simulink model "pato4CM00_plantModel"  (R2017b)
settings: Solver=FixedStepDiscrete  StartTime=0.0  StopTime=1.8  FixedStep=1/2048  RelTol=1e-3  EnableMultiTasking=on
settings Model: ExtModeAutoUpdateStatusClock=off  Creator=root  LastModifiedBy=Job
settings DataIOCC: SaveFormat=Array  SignalLoggingSaveFormat=ModelDataLogs
settings OptimizationCC: ExpressionDepthLimit=2147483647  InitFltsAndDblsToZero=on  LifeSpan=inf
settings DebuggingCC: UnderspecifiedInitializationDetection=Classic  MergeDetectMultiDrivingBlocksExec=none  SolverPrmCheckMsg=warning  FcnCallInpInsideContextMsg=warning  AllowSymbolicDim=off  StateNameClashWarn=warning  SFUnexpectedBacktrackingDiag=warning  SFNoUnconditionalDefaultTransitionDiag=warning  SFExecutionAtInitializationDiag=none
settings HardwareCC: ProdBitPerPointer=32  ProdBitPerSizeT=32  ProdBitPerPtrDiffT=32  ProdLargestAtomicFloat=None  ProdIntDivRoundTo=Undefined  ProdEndianess=Unspecified  ProdWordSize=32  ProdHWDeviceType=32-bit Generic
settings ModelReferenceCC: PropagateSignalLabelsOutOfModel=off
settings RTWCC: SystemTargetFile=ectarget.tlc  MakeCommand="make_rtw OPTS=\"-DNETIF_ID=2\""  TemplateMakefile=ec_unix.tmf  Description=EtherCAT Real-Time Target for SOEM (IME Technologies 2008)
settings CodeAppCC: StateflowObjectComments=on
settings GRTTargetCC: TargetLangStandard=C89/C90 (ANSI)  GeneratePreprocessorConditionals=Disable all  CombineOutputUpdateFcns=off  GRTInterface=on  UseToolchainInfoCompliant=off  ExtMode=on
settings ConfigComp: CovMetricSettings=dw  CovHtmlReporting=on  CovSaveCumulativeToWorkspaceVar=on  CovSaveSingleToWorkspaceVar=on  CovExternalEMLEnable=off  CovSFcnEnable=off

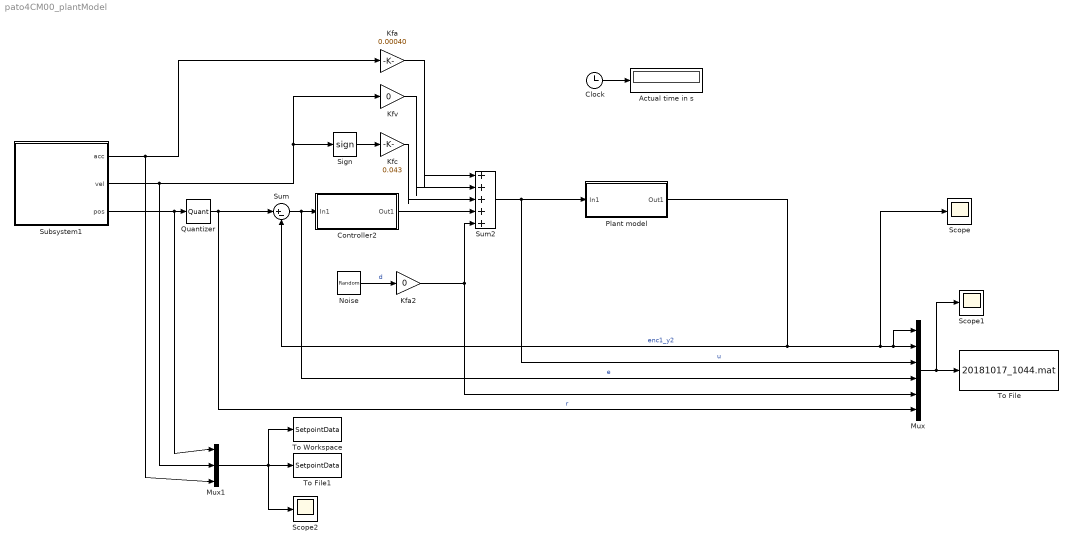
== system pato4CM00_plantModel ==
  Actual time in s : Display
  Clock : Clock
  Controller2 : Subsystem
  Kfa : Gain  Gain=0.00040  SaturateOnIntegerOverflow=on  OutDataTypeStr=Inherit: Same as input  ParamDataTypeStr=Inherit: Same as input
  Kfa2 : Gain  Gain=0  SaturateOnIntegerOverflow=on  OutDataTypeStr=Inherit: Same as input  ParamDataTypeStr=Inherit: Same as input
  Kfc : Gain  Gain=0.043  SaturateOnIntegerOverflow=on  OutDataTypeStr=Inherit: Same as input  ParamDataTypeStr=Inherit: Same as input
  Kfv : Gain  Gain=0  SaturateOnIntegerOverflow=on  OutDataTypeStr=Inherit: Same as input  ParamDataTypeStr=Inherit: Same as input
  Mux : Mux  Inputs=6
  Mux1 : Mux  Inputs=3
  Noise : RandomNumber  Variance=0.1  SampleTime=0
  Plant model : Subsystem
  Quantizer : Quantizer  QuantizationInterval=(2*pi)/(500*4)
  Scope : Scope
  Scope1 : Scope
  Scope2 : Scope
  Sign : Signum
  Subsystem1 : Subsystem  mask(Ref3){}
      settings: OpenFcn=r3g_main
      mask Display: disp('Ref3');
  Sum : Sum  Inputs=|+-  SaturateOnIntegerOverflow=on  InputSameDT=on  OutDataTypeStr=Inherit: Same as first input
  Sum2 : Sum  Description=sumff  Inputs=|+++++  SaturateOnIntegerOverflow=on  InputSameDT=on  OutDataTypeStr=Inherit: Same as first input
  To File : ToFile  Filename=20181017_1044.mat
  To File1 : ToFile  Filename=SetpointData  SaveFormat=Timeseries
  To Workspace : ToWorkspace  VariableName=SetpointData  SaveFormat=Timeseries  SampleTime=-1
  wires:
  Subsystem1/1(acc) -> Mux1/3, Kfa/1
  Sum/1 -> Controller2/1(In1), Mux/4  "e"
  Sign/1 -> Kfc/1
  Kfc/1 -> Sum2/3
  Kfv/1 -> Sum2/2
  Kfa/1 -> Sum2/1
  Sum2/1 -> Plant model/1(In1), Mux/3  "u"
  Subsystem1/3(pos) -> Mux1/1, Quantizer/1
  Subsystem1/2(vel) -> Mux1/2, Kfv/1, Sign/1
  Clock/1 -> Actual time in s/1
  Controller2/1(Out1) -> Sum2/4
  Quantizer/1 -> Sum/1, Mux/6  "r"
  Plant model/1(Out1) -> Sum/2, Mux/1, Mux/2, Scope/1  "enc1_y2"
  Mux/1 -> Scope1/1, To File/1
  Kfa2/1 -> Sum2/5, Mux/5
  Noise/1 -> Kfa2/1  "d"
  Mux1/1 -> To Workspace/1, Scope2/1, To File1/1

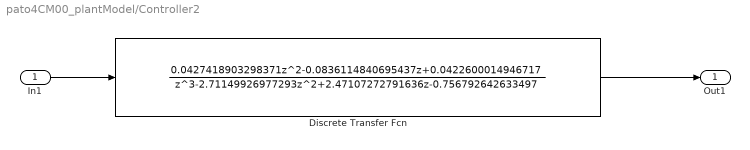
== system pato4CM00_plantModel/Controller2 ==
  In1 : Inport
  Discrete Transfer Fcn : DiscreteTransferFcn  Numerator=[0 0.0427418903298371 -0.0836114840695437 0.0422600014946717]  Denominator=[1 -2.71149926977293 2.47107272791636 -0.756792642633497]  SampleTime=1/2048
  Out1 : Outport
  wires:
  In1/1 -> Discrete Transfer Fcn/1
  Discrete Transfer Fcn/1 -> Out1/1

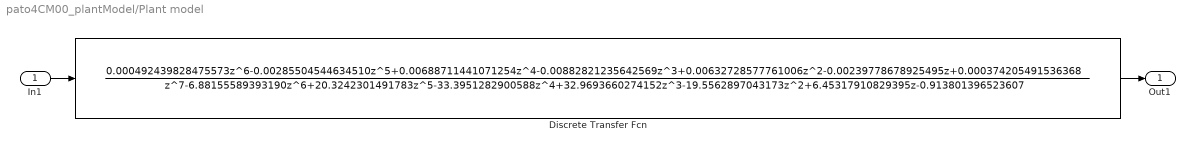
== system pato4CM00_plantModel/Plant model ==
  In1 : Inport
  Discrete Transfer Fcn : DiscreteTransferFcn  Numerator=[0 0.000492439828475573 -0.00285504544634510 0.00688711441071254 -0.00882821235642569 0.00632728577761006 -0.00239778678925495 0.000374205491536368]  Denominator=[1 -6.88155589393190 20.3242301491783 -33.3951282900588 32.9693660274152 -19.5562897043173 6.45317910829395 -0.913801396523607]  SampleTime=1/2048
  Out1 : Outport
  wires:
  Discrete Transfer Fcn/1 -> Out1/1
  In1/1 -> Discrete Transfer Fcn/1

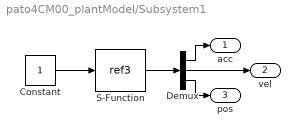
== system pato4CM00_plantModel/Subsystem1 ==
  Constant : Constant
  Demux : Demux  Outputs=3
  S-Function : S-Function  FunctionName=ref3  Parameters=ref_part  SFunctionDeploymentMode=off  EnableBusSupport=off
      settings: OpenFcn=global ref_part; r3g_main
  acc : Outport
  vel : Outport  Port=2
  pos : Outport  Port=3
  wires:
  Constant/1 -> S-Function/1
  S-Function/1 -> Demux/1
  Demux/1 -> acc/1
  Demux/2 -> vel/1
  Demux/3 -> pos/1
